simulink model "dzhan"  (R2024b)
settings: Solver=VariableStepAuto  StartTime=0.0  StopTime=t_f  RelTol=1e-5
undefined symbols (not defined in the file): inertia, vehicle_ornt_0, vehicle_spin_0
settings Model: Creator=yevge  LastModifiedBy=yevge

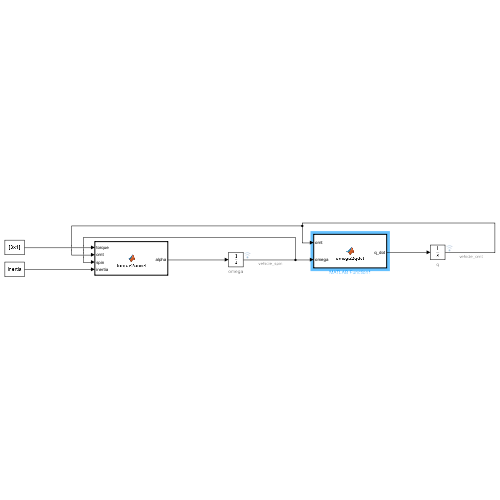
[thumbnail: Simulink's stored preview of the top-level diagram]
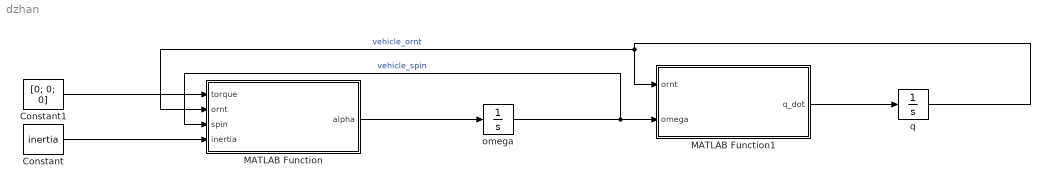
== system dzhan ==
  Constant : Constant  Value=inertia
  Constant1 : Constant  Value=[0; 0; 0]  VectorParams1D=off
  MATLAB Function : MATLAB Function  TreatAsAtomicUnit=on
  MATLAB Function1 : MATLAB Function  TreatAsAtomicUnit=on
  omega : Integrator  InitialCondition=vehicle_spin_0
  q : Integrator  InitialCondition=vehicle_ornt_0
  wires:
  MATLAB Function/1(alpha) -> omega/1
  q/1 -> MATLAB Function1/1(ornt), MATLAB Function/2(ornt)  "vehicle_ornt"
  omega/1 -> MATLAB Function/3(spin), MATLAB Function1/2(omega)  "vehicle_spin"
  MATLAB Function1/1(q_dot) -> q/1
  Constant/1 -> MATLAB Function/4(inertia)
  Constant1/1 -> MATLAB Function/1(torque)

== matlab function dzhan/MATLAB Function1 ==
  data: ornt input; omega input; q_dot output
function q_dot = omega2qdot(ornt, omega)
    q_dot = 0.5 * quatmultiply(ornt', [0 omega'])';
end

== matlab function dzhan/MATLAB Function ==
  data: torque input; alpha output; ornt input; spin input; inertia input
function alpha = torque2accel(torque, ornt, spin, inertia)
    direction = quat2dcm(ornt');
    inertia_global = direction * inertia * direction.';
    alpha = inertia_global \ (torque - cross(spin, inertia_global*spin));
end
